simulink model "BMS"  (R2022b)
settings: Solver=VariableStepAuto  StartTime=0.0  StopTime=10.0  RelTol=1e-3
undefined symbols (not defined in the file): BMS_mode
(part 2 of 2)

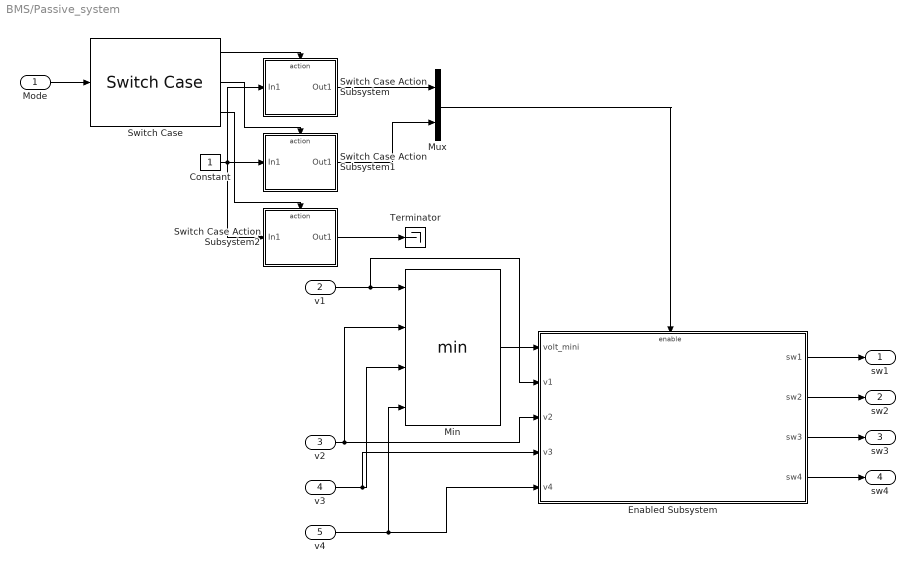
== system BMS/Passive_system ==
  Mode : Inport
  v1 : Inport  Port=2
  v2 : Inport  Port=3
  v3 : Inport  Port=4
  v4 : Inport  Port=5
  Constant : Constant
  Enabled Subsystem : Subsystem  TreatAsAtomicUnit=on
  Min : MinMax  Inputs=4
  Mux : Mux  Inputs=2
  Switch Case : SwitchCase  CaseConditions=[BMS_mode.off,BMS_mode.charging,BMS_mode.discharging]  ShowDefaultCase=off
  Switch Case Action Subsystem : Subsystem  TreatAsAtomicUnit=on
  Switch Case Action Subsystem1 : Subsystem  TreatAsAtomicUnit=on
  Switch Case Action Subsystem2 : Subsystem  TreatAsAtomicUnit=on
  Terminator : Terminator
  sw1 : Outport
  sw2 : Outport  Port=2
  sw3 : Outport  Port=3
  sw4 : Outport  Port=4
  wires:
  v3/1 -> Enabled Subsystem/4(v3), Min/3
  v1/1 -> Enabled Subsystem/2(v1), Min/1
  Mode/1 -> Switch Case/1
  Switch Case Action Subsystem1/1(Out1) -> Mux/2
  Mux/1 -> Enabled Subsystem/Enable
  Switch Case/1 -> Switch Case Action Subsystem/Action
  Switch Case Action Subsystem/1(Out1) -> Mux/1
  Switch Case/2 -> Switch Case Action Subsystem1/Action
  Switch Case/3 -> Switch Case Action Subsystem2/Action
  Switch Case Action Subsystem2/1(Out1) -> Terminator/1
  Constant/1 -> Switch Case Action Subsystem2/1(In1), Switch Case Action Subsystem1/1(In1), Switch Case Action Subsystem/1(In1)
  v2/1 -> Enabled Subsystem/3(v2), Min/2
  v4/1 -> Min/4, Enabled Subsystem/5(v4)
  Min/1 -> Enabled Subsystem/1(volt_mini)
  Enabled Subsystem/2(sw2) -> sw2/1
  Enabled Subsystem/1(sw1) -> sw1/1
  Enabled Subsystem/4(sw4) -> sw4/1
  Enabled Subsystem/3(sw3) -> sw3/1

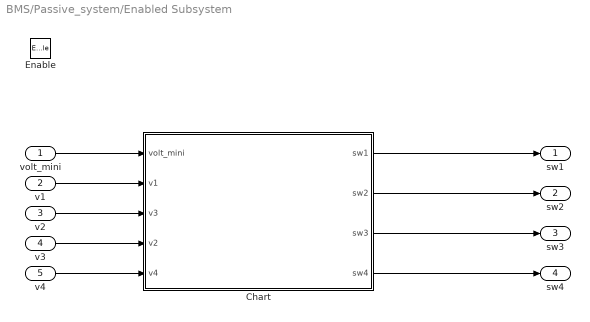
== system BMS/Passive_system/Enabled Subsystem ==
  volt_mini : Inport
  v1 : Inport  Port=2
  v2 : Inport  Port=3
  v3 : Inport  Port=4
  v4 : Inport  Port=5
  Enable : EnablePort
  Chart : Stateflow chart  TreatAsAtomicUnit=on
      settings: PortSchema="{\"entries\":[{\"content\":{\"sides\":[{\"content\":{\"connectorIds\":[\"In1\",\"In2\",\"In3\",\"In4\",\"In5\"]},\"type\":\"ConnectorPlacement.EquallySpacedRectSide\",\"uuid\":\"f29a8cda-8803-475f-abd3-4e4339aba25e\"},{\"content\":{\"connectorIds\":[\"Out2\",\"Out3\",\"Out1\",\"Out4\"],\"side\":\"RIGHT\"},\"type\":\"ConnectorPlacement.EquallySpacedRectSide\",\"uuid\":\"0598b39c-caa4-4adf-8d5c-28c07f0296f4\"},{\"content\":{\"connectorIds\":[],\"side\":\"TOP\"},\"type\":\"ConnectorPlacement.EquallySpacedRectSide\",\"uuid\":\"9f38f119-9f27-4a8e-b2cb-7c7e66af6571\"},{\"content\":{\"connectorIds\":[],\"side\":\"BOTTOM\"},\"type\":\"ConnectorPlacement.EquallySpacedRectSide\",\"uuid\":\"32b45aed-3993-4991-a8ea-fcd5247e15e7\"}]},\"type\":\"ConnectorPlacement.EquallySpacedConnector\",\"uuid\":\"c85bfddf-40ea-4a5b-9c2d-94a149e11b52\"}],\"packageUris\":[\"http://schema.mathworks.com/mf0/Connector/R2020b\"],\"version\":\"1.0\"}"
  sw1 : Outport
  sw2 : Outport  Port=2
  sw3 : Outport  Port=3
  sw4 : Outport  Port=4
  wires:
  volt_mini/1 -> Chart/1(volt_mini)
  Chart/2(sw1) -> sw1/1
  Chart/3(sw2) -> sw2/1
  Chart/1(sw3) -> sw3/1
  Chart/4(sw4) -> sw4/1
  v1/1 -> Chart/2(v1)
  v2/1 -> Chart/3(v3)
  v3/1 -> Chart/4(v2)
  v4/1 -> Chart/5(v4)

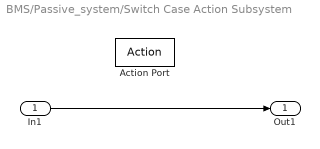
== system BMS/Passive_system/Switch Case Action Subsystem ==
  In1 : Inport
  Action Port : ActionPort  ActionPortLabel=case [ off ]:
  Out1 : Outport
  wires:
  In1/1 -> Out1/1

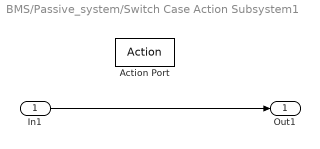
== system BMS/Passive_system/Switch Case Action Subsystem1 ==
  In1 : Inport
  Action Port : ActionPort  ActionPortLabel=case [ charging ]:
  Out1 : Outport
  wires:
  In1/1 -> Out1/1

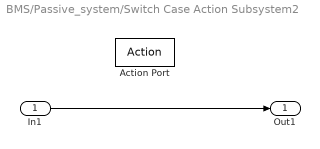
== system BMS/Passive_system/Switch Case Action Subsystem2 ==
  In1 : Inport
  Action Port : ActionPort  ActionPortLabel=case [ discharging ]:
  Out1 : Outport
  wires:
  In1/1 -> Out1/1

== stateflow chart BMS/Passive_system/Enabled Subsystem/Chart ==
  (default) -> (junction 20)
  (junction 20) -> (junction 21) [order 1] : [(volt_mini==v1) ]
  (junction 20) -> (junction 181) [order 2]
  (junction 21) -> (junction 29) : {sw2=1; sw3=1; sw4=1;}
  (junction 181) -> (junction 182) [order 1] : [ (volt_mini==v1)  && ( v2 == (v1 +0.1) ) ]
  (junction 181) -> (junction 22) [order 2]
  (junction 182) -> (junction 183) : {sw2=0;}
  (junction 22) -> (junction 23) [order 1] : [(volt_mini==v1)  && ( v3  == (v1 +0.1) )]
  (junction 22) -> (junction 24) [order 2]
  (junction 23) -> (junction 28) : { sw3=0;}
  (junction 24) -> (junction 25) [order 1] : [(volt_mini==v1)  && ( v4 == (v1 +0.1) )]
  (junction 24) -> (junction 26) [order 2]
  (junction 25) -> (junction 27) : {sw4=0;}
  (junction 27) -> (junction 26)
  (junction 28) -> (junction 27)
  (junction 183) -> (junction 28)
  (junction 29) -> (junction 183)
  (junction 26) -> (junction 48)
  (junction 48) -> (junction 44) [order 1] : [(volt_mini==v2)]
  (junction 48) -> (junction 190) [order 2]
  (junction 44) -> (junction 64) : {sw1=1; sw3=1; sw4=1;}
  (junction 190) -> (junction 191) [order 2] : [(volt_mini==v2)  &&  (v1 == (v2 +0.1) )]
  (junction 191) -> (junction 192) : {sw1=0;}
  (junction 190) -> (junction 42) [order 1]
  (junction 42) -> (junction 43) [order 1] : [(volt_mini==v2)  && ( v3 == (v2 +0.1) )]
  (junction 42) -> (junction 38) [order 2]
  (junction 43) -> (junction 49) : { sw3=0;}
  (junction 38) -> (junction 39) [order 1] : [(volt_mini==v2)  &&  (v4 == (v2 +0.1) )]
  (junction 38) -> (junction 45) [order 2]
  (junction 39) -> (junction 40) : {sw4=0;}
  (junction 64) -> (junction 192)
  (junction 192) -> (junction 49)
  (junction 40) -> (junction 45)
  (junction 49) -> (junction 40)
  (junction 45) -> (junction 120)
  (junction 120) -> (junction 111) [order 1] : [(volt_mini==v3)]
  (junction 120) -> (junction 199) [order 2]
  (junction 111) -> (junction 96) : {sw1=1; sw2=1; sw4=1;}
  (junction 199) -> (junction 200) [order 1] : [(volt_mini==v3)  && ( v1 == (v3 +0.1) )]
  (junction 200) -> (junction 201) : {sw1=0;}
  (junction 199) -> (junction 117) [order 2]
  (junction 117) -> (junction 116) [order 1] : [(volt_mini==v3)  && ( v2 == (v3 +0.1) )]
  (junction 117) -> (junction 113) [order 2]
  (junction 116) -> (junction 114) : {sw2=0;}
  (junction 113) -> (junction 97) [order 1] : [(volt_mini==v3)  && ( v4 == (v3 +0.1) )]
  (junction 113) -> (junction 109) [order 2]
  (junction 97) -> (junction 105) : {sw4=0;}
  (junction 201) -> (junction 114)
  (junction 96) -> (junction 201)
  (junction 114) -> (junction 105)
  (junction 105) -> (junction 109)
  (junction 109) -> (junction 208)
  (junction 208) -> (junction 209) [order 1] : [(volt_mini==v4)]
  (junction 208) -> (junction 144) [order 2]
  (junction 209) -> (junction 210) : {sw1=1; sw2=1; sw3=1;}
  (junction 144) -> (junction 139) [order 1] : [(volt_mini==v4)  && ( v1 == (v4 +0.1) ) ]
  (junction 144) -> (junction 134) [order 2]
  (junction 139) -> (junction 138) : {sw1=0;}
  (junction 134) -> (junction 132) [order 1] : [(volt_mini==v4)  && ( v2 == (v4 +0.1) )]
  (junction 134) -> (junction 143) [order 2]
  (junction 132) -> (junction 122) : { sw2=0;}
  (junction 143) -> (junction 131) [order 1] : [(volt_mini==v4)  && ( v3 == (v4 +0.1) )]
  (junction 143) -> (junction 140) [order 2]
  (junction 131) -> (junction 126) : {sw3=0;}
  (junction 126) -> (junction 140)
  (junction 122) -> (junction 126)
  (junction 210) -> (junction 122)
  (junction 138) -> (junction 210)
  (junction 140) -> (junction 145)
  data: sw3 output; volt_mini input; sw1 output; sw2 output; sw4 output; v1 input; v3 input; v2 input; v4 input
